simulink model "SVPWM"  (R2022a)
settings: Solver=VariableStepAuto  StartTime=0.0  StopTime=1  RelTol=1e-3
libraries: spsPLLLib x1, simulink x1, spspowerguiLib x1
settings Model: Creator=nikos  LastModifiedBy=nikos

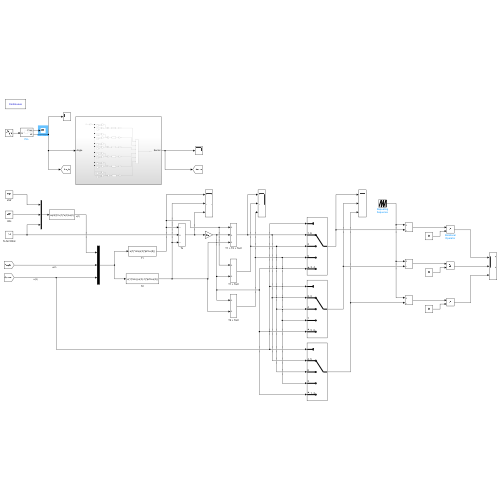
[thumbnail: Simulink's stored preview of the top-level diagram]
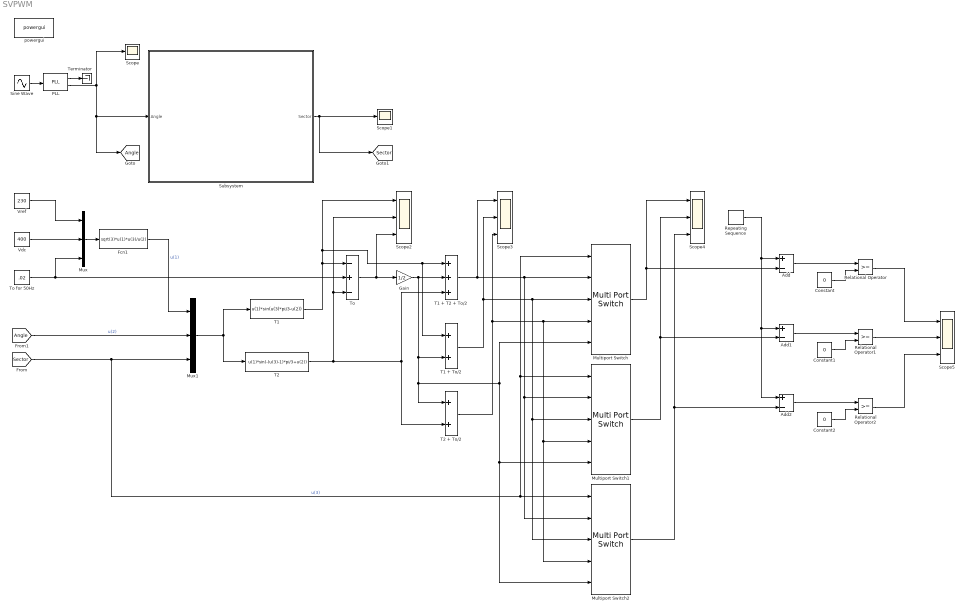
== system SVPWM ==
  Add : Sum  Inputs=+-
  Add1 : Sum  Inputs=+-
  Add2 : Sum  Inputs=+-
  Constant : Constant  Value=0
  Constant1 : Constant  Value=0
  Constant2 : Constant  Value=0
  Fcn1 : Fcn  Expr=sqrt(3)*u(1)*u(3)/u(2)
  Gain : Gain  Gain=1/2
  Multiport Switch : MultiPortSwitch  DataPortOrder=Specify indices  DataPortIndices={[1,6],2,5,[3,4]}  SaturateOnIntegerOverflow=off  InputSameDT=off
  Multiport Switch1 : MultiPortSwitch  DataPortOrder=Specify indices  DataPortIndices={[2,3],4,1,[5,6]}  SaturateOnIntegerOverflow=off  InputSameDT=off
  Multiport Switch2 : MultiPortSwitch  DataPortOrder=Specify indices  DataPortIndices={[4,5],6,3,[1,2]}  SaturateOnIntegerOverflow=off  InputSameDT=off
  Mux : Mux  Inputs=3
  Mux1 : Mux  Inputs=3
  PLL : spsPLLLib/PLL  Fmin=45  Par_Init=[0, 60]  ParK=[180, 3200, 1]  TcD=1e-4  MaxRateChangeFreq=12  FilterCutOffFreq=25  Ts=0  AGC=on
      settings: SourceProductBaseCode=PS
  Relational Operator : RelationalOperator  OutDataTypeStr=boolean  RndMeth=Simplest  InputSameDT=off
  Relational Operator1 : RelationalOperator  OutDataTypeStr=boolean  RndMeth=Simplest  InputSameDT=off
  Relational Operator2 : RelationalOperator  OutDataTypeStr=boolean  RndMeth=Simplest  InputSameDT=off
  Repeating Sequence : simulink/Sources/Repeating Sequence  rep_seq_t=[0 0.001]  rep_seq_y=[0 0.02]
  Scope : Scope
  Scope1 : Scope
  Scope{2..5} (4 alike) : Scope  NumInputPorts=3
  Sine Wave : Sin  Frequency=2*pi*50  SampleTime=0
  Subsystem : Subsystem
  T1 : Fcn  Expr=u(1)*sin(u(3)*pi/3-u(2))
  T1 + T2 + To/2 : Sum  Inputs=+++
  T1 + To/2 : Sum
  T2 : Fcn  Expr=u(1)*sin(-(u(3)-1)*pi/3+u(2))
  T2 + To/2 : Sum
  Terminator : Terminator
  To : Sum  Inputs=-+-
  To for 50Hz : Constant  Value=.02
  Vdc : Constant  Value=400
  Vref : Constant  Value=230
  powergui : spspowerguiLib/powergui  Priority=1  SimulationMode=Continuous  SampleTime=50e-6  frequency=60  Iterations=50  frequencyindice=60  Pbase=100e6  ErrMax=1e-4  UnitsV=kV  UnitsW=MW  buscounter=0  FunctionMessages=off  echomessages=off  EnableUseOfTLC=off  CurrentSourceSwitches=off  DisableSnubberDevices=off  DisableRonSwitches=off  DisableVfSwitches=off  DisplayEquations=off  AutomaticDiscreteSolvers=off  SolverType=Tustin/Backward Euler (TBE)  Interpol=off  ExternalGateDelay=off  methode=off  Ts=100  x0status=blocks  SPID=on  SwTol=0  HookPort=off  NonlinearTolerance=1e-4  nMaxIteration=100  ContinueOnMaxIteration=off  RestoreLinks=warning  ResistiveCurrentMeasurement=off  Frange=[0:2:500]  Ylog=off  Xlog=on  ShowGrid=off  save=off  variable=ZData  structure=0  ZoomFFT=off  StartTime=0.0  cycles=1  DisplayStyle=1  fundamental=60  FreqAxis=off  MaxFrequency=1000  frequencyindicesteady=1  RmsSteady=1  display=off
  tag scope: Angle=global, Sector=global
  wires:
  Vdc/1 -> Mux/2
  Vref/1 -> Mux/1
  To for 50Hz/1 -> To/2, Mux/3
  Sine Wave/1 -> PLL/1
  PLL/2 -> [Angle], Subsystem/1(Angle), Scope/1
  Subsystem/1(Sector) -> [Sector], Scope1/1
  Mux/1 -> Fcn1/1
  [Angle] -> Mux1/2  "u(2)"
  [Sector] -> Multiport Switch2/1, Multiport Switch/1, Multiport Switch1/1, Mux1/3  "u(3)"
  Fcn1/1 -> Mux1/1  "u(1)"
  Mux1/1 -> T2/1, T1/1
  T1/1 -> To/1, T1 + To/2/1, T1 + T2 + To/2/1, Scope2/1
  To/1 -> Scope2/3, Gain/1
  Gain/1 -> T1 + To/2/2, T2 + To/2/1, Multiport Switch2/5, Multiport Switch1/5, Multiport Switch/5, T1 + T2 + To/2/2
  T1 + T2 + To/2/1 -> Multiport Switch2/2, Multiport Switch1/2, Multiport Switch/2, Scope3/1
  T1 + To/2/1 -> Multiport Switch2/3, Multiport Switch1/3, Multiport Switch/3, Scope3/2
  T2 + To/2/1 -> Multiport Switch2/4, Multiport Switch1/4, Multiport Switch/4, Scope3/3
  T2/1 -> Scope2/2, To/3, T2 + To/2/2, T1 + T2 + To/2/3
  Multiport Switch1/1 -> Scope4/2, Add1/2
  Multiport Switch/1 -> Add/2, Scope4/1
  Multiport Switch2/1 -> Scope4/3, Add2/2
  Repeating Sequence/1 -> Add2/1, Add1/1, Add/1
  Add/1 -> Relational Operator/1
  Constant/1 -> Relational Operator/2
  Constant1/1 -> Relational Operator1/2
  Add1/1 -> Relational Operator1/1
  Add2/1 -> Relational Operator2/1
  Constant2/1 -> Relational Operator2/2
  Relational Operator/1 -> Scope5/1
  Relational Operator1/1 -> Scope5/2
  Relational Operator2/1 -> Scope5/3
  PLL/1 -> Terminator/1

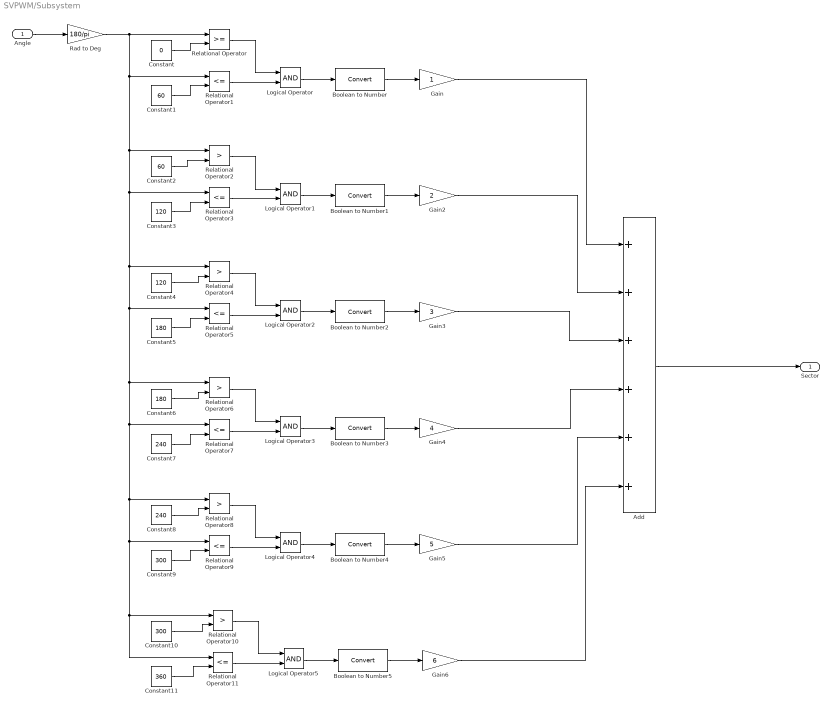
== system SVPWM/Subsystem ==
  Angle : Inport
  Add : Sum  Inputs=++++++
  Boolean to Number{,1..5} (6 alike) : DataTypeConversion  SaturateOnIntegerOverflow=off  RndMeth=Floor
  Constant : Constant  Value=0
  Constant1 : Constant  Value=60
  Constant10 : Constant  Value=300
  Constant11 : Constant  Value=360
  Constant2 : Constant  Value=60
  Constant3 : Constant  Value=120
  Constant4 : Constant  Value=120
  Constant5 : Constant  Value=180
  Constant6 : Constant  Value=180
  Constant7 : Constant  Value=240
  Constant8 : Constant  Value=240
  Constant9 : Constant  Value=300
  Gain : Gain
  Gain2 : Gain  Gain=2
  Gain3 : Gain  Gain=3
  Gain4 : Gain  Gain=4
  Gain5 : Gain  Gain=5
  Gain6 : Gain  Gain=6
  Logical Operator{,1..5} (6 alike) : Logic  AllPortsSameDT=off  OutDataTypeStr=boolean
  Rad to Deg : Gain  Gain=180/pi
  Relational Operator : RelationalOperator  OutDataTypeStr=boolean  RndMeth=Simplest  InputSameDT=off
  Relational Operator{1,3,5,7,9,11} (6 alike) : RelationalOperator  Operator=<=  OutDataTypeStr=boolean  RndMeth=Simplest  InputSameDT=off
  Relational Operator{2,4,6,8,10} (5 alike) : RelationalOperator  Operator=>  OutDataTypeStr=boolean  RndMeth=Simplest  InputSameDT=off
  Sector : Outport
  wires:
  Angle/1 -> Rad to Deg/1
  Constant/1 -> Relational Operator/2
  Constant1/1 -> Relational Operator1/2
  Relational Operator/1 -> Logical Operator/1
  Relational Operator1/1 -> Logical Operator/2
  Logical Operator/1 -> Boolean to Number/1
  Boolean to Number/1 -> Gain/1
  Boolean to Number1/1 -> Gain2/1
  Logical Operator1/1 -> Boolean to Number1/1
  Relational Operator3/1 -> Logical Operator1/2
  Relational Operator2/1 -> Logical Operator1/1
  Constant3/1 -> Relational Operator3/2
  Constant2/1 -> Relational Operator2/2
  Constant4/1 -> Relational Operator4/2
  Constant5/1 -> Relational Operator5/2
  Relational Operator4/1 -> Logical Operator2/1
  Relational Operator5/1 -> Logical Operator2/2
  Logical Operator2/1 -> Boolean to Number2/1
  Boolean to Number2/1 -> Gain3/1
  Boolean to Number3/1 -> Gain4/1
  Logical Operator3/1 -> Boolean to Number3/1
  Relational Operator7/1 -> Logical Operator3/2
  Relational Operator6/1 -> Logical Operator3/1
  Constant7/1 -> Relational Operator7/2
  Constant6/1 -> Relational Operator6/2
  Constant8/1 -> Relational Operator8/2
  Constant9/1 -> Relational Operator9/2
  Relational Operator8/1 -> Logical Operator4/1
  Relational Operator9/1 -> Logical Operator4/2
  Logical Operator4/1 -> Boolean to Number4/1
  Boolean to Number4/1 -> Gain5/1
  Boolean to Number5/1 -> Gain6/1
  Logical Operator5/1 -> Boolean to Number5/1
  Relational Operator11/1 -> Logical Operator5/2
  Relational Operator10/1 -> Logical Operator5/1
  Constant11/1 -> Relational Operator11/2
  Constant10/1 -> Relational Operator10/2
  Rad to Deg/1 -> Relational Operator/1, Relational Operator10/1, Relational Operator11/1, Relational Operator9/1, Relational Operator8/1, Relational Operator7/1, Relational Operator6/1, Relational Operator5/1, Relational Operator4/1, Relational Operator3/1, Relational Operator2/1, Relational Operator1/1
  Gain/1 -> Add/1
  Gain2/1 -> Add/2
  Gain3/1 -> Add/3
  Gain4/1 -> Add/4
  Gain5/1 -> Add/5
  Gain6/1 -> Add/6
  Add/1 -> Sector/1
